simulink model "WindEmulatorDriveSim"  (R2021a)
settings: Solver=FixedStepDiscrete  StartTime=0.0  StopTime=inf  FixedStep=0.002  RelTol=1e-3
values from neighbouring files (symbols this model uses):
  ctrlModeSpeed = logical(false)    [initStep4.m]
  ctrlModeTorque = logical(true)    [initStep4.m]
  StatusWord = bitset(StatusWord,16)    [VFD_StatusWord.m]
undefined symbols (not defined in the file or in its folder): Gen_REF2_Max, Gen_SpeedScaling, Motor_SpeedScaling, Motor_TorqueScaling
libraries: slrealtimeethercatlib x21, simulink x4
settings Model: SimulationMode=external  Creator=SWEPT  LastModifiedBy=Johannes
settings SolverCC: ConcurrentTasks=on  PositivePriorityOrder=on
settings OptimizationCC: BlockReduction=off  OptimizeBlockIOStorage=off
settings DebuggingCC: TasksWithSamePriorityMsg=none
settings HardwareCC: ProdBitPerLong=64  ProdLongLongMode=on  ProdHWDeviceType=Intel->x86-64 (Linux 64)
settings RTWCC: Description=Simulink Real-Time  SystemTargetFile=slrealtime.tlc  TemplateMakefile=slrealtime_default_tmf  RTWVerbose=off  Toolchain=Simulink Real-Time Toolchain  BuildConfiguration=Faster Runs  CodeExecutionProfiling=on  TargetLang=C++

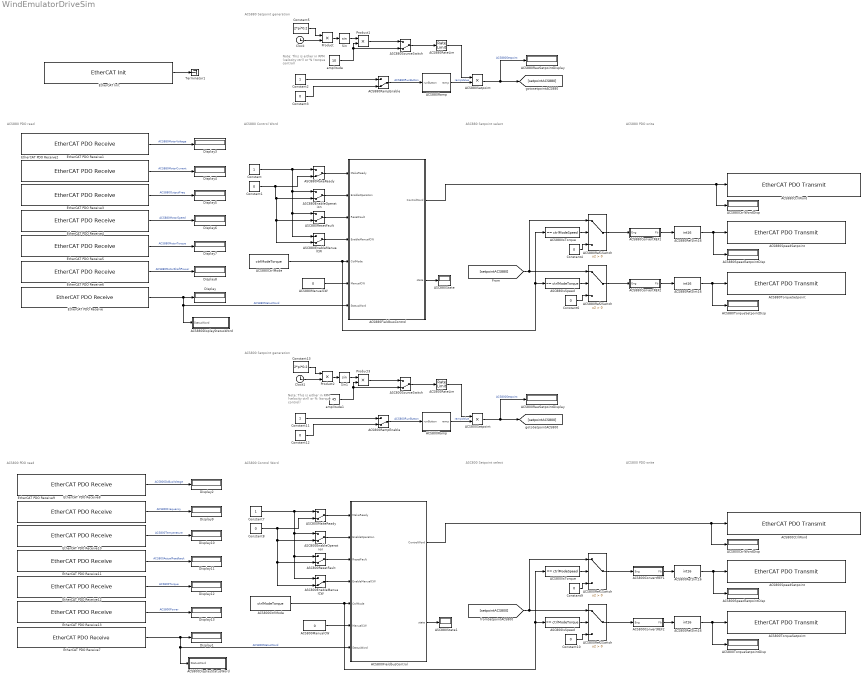
== system WindEmulatorDriveSim ==
  note: ACS880 Setpoint generation
  note: ACS880 PDO write
  note: ASC880 Setpoint select
  note: Note: This is either in RPM (velocity ctrl) or % (torque control)
  note: ACS880 Control Word
  note: ACS880 PDO read
  note: ACS800 PDO read
  note: ACS800 Control Word
  note: ASC800 Setpoint select
  note: ACS800 PDO write
  note: ACS800 Setpoint generation
  note: Note: This is either in RPM (velocity ctrl) or % (torque control)
  ACS800ConvertREF1 : Subsystem  mask{EngineeringValue=Gen_SpeedScaling, FieldbusValue=20000}
      mask prompts: EngineeringValue "Engineering units nominal value:"; FieldbusValue "Fieldbus nominal value:"
  ACS800ConvertREF2 : Subsystem  mask{EngineeringValue=Gen_REF2_Max, FieldbusValue=10000}
      mask prompts: EngineeringValue "Engineering units nominal value:"; FieldbusValue "Fieldbus nominal value:"
  ACS800CtrlMode : Constant  Value=ctrlModeTorque  OutDataTypeStr=boolean
  ACS800CtrlWord : slrealtimeethercatlib/EtherCAT PDO Transmit  Priority=3  sig_name=Drive 2 (RECA-01 r2.07 and ACS800).RxPDO 1.ControlWord (Transparent)  sig_offset=384  sig_type=uint16  type_size=16  sig_dim=1  device_id=0  sample_time=0.002000
      settings: SourceProductBaseCode=XP
  ACS800CtrlWordDisp : Display
  ACS800DisplayStatusWord : Subsystem
  ACS800FieldbusControl : Subsystem
  ACS800IsTorque : simulink/Logic and Bit Operations/Compare To Constant  relop===  const=ctrlModeSpeed  OutDataTypeStr=boolean
  ACS800ManualCW : Constant  Value=0  OutDataTypeStr=uint16
  ACS800Ramp : Stateflow chart  TreatAsAtomicUnit=on
  ACS800RampEnable : ManualSwitch  CurrentSetting=0
  ACS800RateLim : RateLimiter  RisingSlewLimit=10000  FallingSlewLimit=-10000  SampleTimeMode=inherited
  ACS800RawSetpointDisplay : Display
  ACS800Ref1Int16 : DataTypeConversion  OutDataTypeStr=int16
  ACS800Ref1Switch : Switch  Criteria=u2 > Threshold
  ACS800Ref2Int16 : DataTypeConversion  OutDataTypeStr=int16
  ACS800Ref2Switch : Switch  Criteria=u2 > Threshold
  ACS800Setpoint : Product
  ACS800SpeedSetpoint : slrealtimeethercatlib/EtherCAT PDO Transmit  Priority=3  sig_name=Drive 2 (RECA-01 r2.07 and ACS800).RxPDO 1.REF1 (Speed)  sig_offset=400  sig_type=int16  type_size=16  sig_dim=1  device_id=0  sample_time=0.002000
      settings: SourceProductBaseCode=XP
  ACS800SpeedSetpointDisp : Display
  ACS800TorqueSetpoint : slrealtimeethercatlib/EtherCAT PDO Transmit  Priority=3  sig_name=Drive 2 (RECA-01 r2.07 and ACS800).RxPDO 1.REF2 (Torque)  sig_offset=416  sig_type=int16  type_size=16  sig_dim=1  device_id=0  sample_time=0.002000
      settings: SourceProductBaseCode=XP
  ACS800TorqueSetpointDisp : Display
  ACS880ConvertREF1 : Subsystem  mask{EngineeringValue=Motor_SpeedScaling, FieldbusValue=20000}
      mask prompts: EngineeringValue "Engineering units nominal value:"; FieldbusValue "Fieldbus nominal value:"
  ACS880ConvertREF2 : Subsystem  mask{EngineeringValue=Motor_TorqueScaling, FieldbusValue=10000}
      mask prompts: EngineeringValue "Engineering units nominal value:"; FieldbusValue "Fieldbus nominal value:"
  ACS880CtrlMode : Constant  Value=ctrlModeTorque  OutDataTypeStr=boolean
  ACS880CtrlWord : slrealtimeethercatlib/EtherCAT PDO Transmit  Priority=3  sig_name=Drive 1 (FECA-01 r1.31 and ACS880).RxPDO 1.ABB Drives Control Word  sig_offset=208  sig_type=uint16  type_size=16  sig_dim=1  device_id=0  sample_time=0.002000
      settings: SourceProductBaseCode=XP
  ACS880CtrlWordDisp : Display
  ACS880DisplayStatusWord : Subsystem
  ACS880FieldbusControl : Subsystem
  ACS880IsTorque : simulink/Logic and Bit Operations/Compare To Constant  relop===  const=ctrlModeSpeed  OutDataTypeStr=boolean
  ACS880ManualCW : Constant  Value=0  OutDataTypeStr=uint16
  ACS880Ramp : Stateflow chart  TreatAsAtomicUnit=on
  ACS880RampEnable : ManualSwitch  CurrentSetting=0
  ACS880RateLim : RateLimiter  RisingSlewLimit=10000  FallingSlewLimit=-10000  SampleTimeMode=inherited
  ACS880RawSetpointDisplay : Display
  ACS880Ref1Int16 : DataTypeConversion  OutDataTypeStr=int16
  ACS880Ref1Switch : Switch  Criteria=u2 > Threshold
  ACS880Ref2Int16 : DataTypeConversion  OutDataTypeStr=int16
  ACS880Ref2Switch : Switch  Criteria=u2 > Threshold
  ACS880Setpoint : Product
  ACS880SpeedSetpoint : slrealtimeethercatlib/EtherCAT PDO Transmit  Priority=3  sig_name=Drive 1 (FECA-01 r1.31 and ACS880).RxPDO 1.ABB Drives REF1  sig_offset=224  sig_type=int16  type_size=16  sig_dim=1  device_id=0  sample_time=0.002000
      settings: SourceProductBaseCode=XP
  ACS880SpeedSetpointDisp : Display
  ACS880TorqueSetpoint : slrealtimeethercatlib/EtherCAT PDO Transmit  Priority=3  sig_name=Drive 1 (FECA-01 r1.31 and ACS880).RxPDO 1.ABB Drives REF2  sig_offset=240  sig_type=int16  type_size=16  sig_dim=1  device_id=0  sample_time=0.002000
      settings: SourceProductBaseCode=XP
  ACS880TorqueSetpointDisp : Display
  ASC800EnableManualCW : ManualSwitch  CurrentSetting=0
  ASC800EnableOperation : ManualSwitch  CurrentSetting=0
  ASC800IsSpeed : simulink/Logic and Bit Operations/Compare To Constant  relop===  const=ctrlModeTorque  OutDataTypeStr=boolean
  ASC800MakeReady : ManualSwitch  CurrentSetting=0
  ASC800ResetFault : ManualSwitch  CurrentSetting=0
  ASC800SourceSwitch : ManualSwitch  CurrentSetting=0
  ASC880EnableManualCW : ManualSwitch  CurrentSetting=0
  ASC880EnableOperation : ManualSwitch  CurrentSetting=0
  ASC880IsSpeed : simulink/Logic and Bit Operations/Compare To Constant  relop===  const=ctrlModeTorque  OutDataTypeStr=boolean
  ASC880MakeReady : ManualSwitch  CurrentSetting=0
  ASC880ResetFault : ManualSwitch  CurrentSetting=0
  ASC880SourceSwitch : ManualSwitch  CurrentSetting=0
  ASC880State : Display
  ASC880State1 : Display
  Clock : Clock
  Clock1 : Clock
  Constant{,2,7,11} (4 alike) : Constant
  Constant{1,3..4,6,8..10,12} (8 alike) : Constant  Value=0
  Constant13 : Constant  Value=2*pi*0.2
  Constant5 : Constant  Value=2*pi*0.2
  Display{,1..13} (14 alike) : Display
  EtherCAT Init : slrealtimeethercatlib/EtherCAT Init  Priority=0  config_file=D:\src\sandia\ptoTest\WindEmulatorFiles\ethercat\WindTurbineEmulator-03-24-2022.xml  device_id=0  pci_bus=0  pci_slot=0  pci_function=0  portnum=1  initstate=2  dctuning=0  enaDebug=0  enaDC=on  errLink=off  masterDbg=off  stateChgDbg=off  baseClock=off  masterCfg=off  logFile='c:\dbglog.txt'  sample_time=0.002000  DCMode=0
      settings: SourceProductBaseCode=XP
  EtherCAT PDO Receive : slrealtimeethercatlib/EtherCAT PDO Receive  Priority=2  sig_name=Drive 1 (FECA-01 r1.31 and ACS880).TxPDO 1.ABB Drives Status Word  sig_offset=208  sig_type=uint16  type_size=16  sig_dim=1  device_id=0  sample_time=0.002000
      settings: SourceProductBaseCode=XP
  EtherCAT PDO Receive1 : slrealtimeethercatlib/EtherCAT PDO Receive  Priority=2  sig_name=Drive 1 (FECA-01 r1.31 and ACS880).TxPDO 6.Calculated motor voltage  sig_offset=304  sig_type=int16  type_size=16  sig_dim=1  device_id=0  sample_time=0.002000
      settings: SourceProductBaseCode=XP
  EtherCAT PDO Receive10 : slrealtimeethercatlib/EtherCAT PDO Receive  Priority=2  sig_name=Drive 2 (RECA-01 r2.07 and ACS800).TxPDO 1.Converter Temperature  sig_offset=496  sig_type=int16  type_size=16  sig_dim=1  device_id=0  sample_time=0.002000
      settings: SourceProductBaseCode=XP
  EtherCAT PDO Receive11 : slrealtimeethercatlib/EtherCAT PDO Receive  Priority=2  sig_name=Drive 2 (RECA-01 r2.07 and ACS800).TxPDO 1.Actual Feedback (Transparent)  sig_offset=400  sig_type=int16  type_size=16  sig_dim=1  device_id=0  sample_time=0.002000
      settings: SourceProductBaseCode=XP
  EtherCAT PDO Receive12 : slrealtimeethercatlib/EtherCAT PDO Receive  Priority=2  sig_name=Drive 2 (RECA-01 r2.07 and ACS800).TxPDO 1.Torque  sig_offset=432  sig_type=int16  type_size=16  sig_dim=1  device_id=0  sample_time=0.002000
      settings: SourceProductBaseCode=XP
  EtherCAT PDO Receive13 : slrealtimeethercatlib/EtherCAT PDO Receive  Priority=2  sig_name=Drive 2 (RECA-01 r2.07 and ACS800).TxPDO 1.Power  sig_offset=448  sig_type=int16  type_size=16  sig_dim=1  device_id=0  sample_time=0.002000
      settings: SourceProductBaseCode=XP
  EtherCAT PDO Receive2 : slrealtimeethercatlib/EtherCAT PDO Receive  Priority=2  sig_name=Drive 1 (FECA-01 r1.31 and ACS880).TxPDO 6.Measured motor current  sig_offset=288  sig_type=int16  type_size=16  sig_dim=1  device_id=0  sample_time=0.002000
      settings: SourceProductBaseCode=XP
  EtherCAT PDO Receive3 : slrealtimeethercatlib/EtherCAT PDO Receive  Priority=2  sig_name=Drive 1 (FECA-01 r1.31 and ACS880).TxPDO 6.Estimated output frequency  sig_offset=272  sig_type=int16  type_size=16  sig_dim=1  device_id=0  sample_time=0.002000
      settings: SourceProductBaseCode=XP
  EtherCAT PDO Receive4 : slrealtimeethercatlib/EtherCAT PDO Receive  Priority=2  sig_name=Drive 1 (FECA-01 r1.31 and ACS880).TxPDO 6.Motor speed used  sig_offset=256  sig_type=int16  type_size=16  sig_dim=1  device_id=0  sample_time=0.002000
      settings: SourceProductBaseCode=XP
  EtherCAT PDO Receive5 : slrealtimeethercatlib/EtherCAT PDO Receive  Priority=2  sig_name=Drive 1 (FECA-01 r1.31 and ACS880).TxPDO 6.Motor torque  sig_offset=320  sig_type=int16  type_size=16  sig_dim=1  device_id=0  sample_time=0.002000
      settings: SourceProductBaseCode=XP
  EtherCAT PDO Receive6 : slrealtimeethercatlib/EtherCAT PDO Receive  Priority=2  sig_name=Drive 1 (FECA-01 r1.31 and ACS880).TxPDO 6.Estimated motor shaft power  sig_offset=336  sig_type=int16  type_size=16  sig_dim=1  device_id=0  sample_time=0.002000
      settings: SourceProductBaseCode=XP
  EtherCAT PDO Receive7 : slrealtimeethercatlib/EtherCAT PDO Receive  Priority=2  sig_name=Drive 2 (RECA-01 r2.07 and ACS800).TxPDO 1.Main StatusWord (Transparent)  sig_offset=384  sig_type=uint16  type_size=16  sig_dim=1  device_id=0  sample_time=0.002000
      settings: SourceProductBaseCode=XP
  EtherCAT PDO Receive8 : slrealtimeethercatlib/EtherCAT PDO Receive  Priority=2  sig_name=Drive 2 (RECA-01 r2.07 and ACS800).TxPDO 1.DC Bus Voltage  sig_offset=480  sig_type=int16  type_size=16  sig_dim=1  device_id=0  sample_time=0.002000
      settings: SourceProductBaseCode=XP
  EtherCAT PDO Receive9 : slrealtimeethercatlib/EtherCAT PDO Receive  Priority=2  sig_name=Drive 2 (RECA-01 r2.07 and ACS800).TxPDO 1.Frequency  sig_offset=464  sig_type=int16  type_size=16  sig_dim=1  device_id=0  sample_time=0.002000
      settings: SourceProductBaseCode=XP
  Product{,1..3} (4 alike) : Product
  Sin : Trigonometry
  Sin1 : Trigonometry
  Terminator1 : Terminator
  amplitude : Constant  Value=10
  amplitude1 : Constant  Value=45
  wires:
  EtherCAT Init/1 -> Terminator1/1
  ASC880EnableOperation/1 -> ACS880FieldbusControl/2(EnableOperation)
  ACS880ManualCW/1 -> ACS880FieldbusControl/6(ManualCW)
  ASC880ResetFault/1 -> ACS880FieldbusControl/3(ResetFault)
  ASC880MakeReady/1 -> ACS880FieldbusControl/1(MakeReady)
  ASC880EnableManualCW/1 -> ACS880FieldbusControl/4(EnableManualCW)
  Constant1/1 -> ASC880EnableManualCW/2, ASC880ResetFault/2, ASC880EnableOperation/2, ASC880MakeReady/2
  Constant/1 -> ASC880EnableManualCW/1, ASC880ResetFault/1, ASC880EnableOperation/1, ASC880MakeReady/1
  ACS880FieldbusControl/2(state) -> ASC880State/1
  EtherCAT PDO Receive1/1 -> Display3/1  "ACS880MotorVoltage"
  EtherCAT PDO Receive2/1 -> Display4/1  "ACS880MotorCurrent"
  EtherCAT PDO Receive3/1 -> Display5/1  "ACS880OutputFreq"
  EtherCAT PDO Receive4/1 -> Display6/1  "ACS880MotorSpeed"
  EtherCAT PDO Receive5/1 -> Display7/1  "ACS880MotorTorque"
  EtherCAT PDO Receive6/1 -> Display8/1  "ACS880MotorShaftPower"
  ACS880RampEnable/1 -> ACS880Ramp/1(runButton)  "ACS880RunButton"
  Constant3/1 -> ACS880RampEnable/2
  Constant2/1 -> ACS880RampEnable/1
  ACS880Ramp/1(ramp) -> ACS880Setpoint/2  "rampValue"
  Clock/1 -> Product/2
  Product/1 -> Sin/1
  Constant5/1 -> Product/1
  ACS880Setpoint/1 -> [setpointACS880], ACS880RawSetpointDisplay/1  "ACS880Setpoint"
  ACS880RateLim/1 -> ACS880Setpoint/1
  ACS880ConvertREF1/1(Fb) -> ACS880Ref1Int16/1
  ACS880Ref1Int16/1 -> ACS880SpeedSetpointDisp/1, ACS880SpeedSetpoint/1
  ACS880Ref2Int16/1 -> ACS880TorqueSetpoint/1, ACS880TorqueSetpointDisp/1
  ACS880ConvertREF2/1(Fb) -> ACS880Ref2Int16/1
  ACS880CtrlMode/1 -> ACS880FieldbusControl/5(CtrlMode), ACS880IsTorque/1, ASC880IsSpeed/1
  EtherCAT PDO Receive/1 -> ACS880DisplayStatusWord/1(StatusWord), ACS880FieldbusControl/7(StatusWord), Display/1  "ACS880StatusWord"
  ACS880IsTorque/1 -> ACS880Ref1Switch/2
  [setpointACS880] -> ACS880Ref1Switch/1, ACS880Ref2Switch/1
  Constant4/1 -> ACS880Ref1Switch/3
  ASC880IsSpeed/1 -> ACS880Ref2Switch/2
  Constant6/1 -> ACS880Ref2Switch/3
  ACS880FieldbusControl/1(ControlWord) -> ACS880CtrlWordDisp/1, ACS880CtrlWord/1
  ACS880Ref1Switch/1 -> ACS880ConvertREF1/1(Eng)
  ACS880Ref2Switch/1 -> ACS880ConvertREF2/1(Eng)
  Sin/1 -> Product1/1
  amplitude/1 -> Product1/2, ASC880SourceSwitch/2
  Product1/1 -> ASC880SourceSwitch/1
  ASC880SourceSwitch/1 -> ACS880RateLim/1
  EtherCAT PDO Receive13/1 -> Display13/1  "ACS800Power"
  EtherCAT PDO Receive11/1 -> Display11/1  "ACS800ActualFeedback"
  EtherCAT PDO Receive9/1 -> Display9/1  "ACS800Frequency"
  EtherCAT PDO Receive12/1 -> Display12/1  "ACS800Torque"
  EtherCAT PDO Receive10/1 -> Display10/1  "ACS800Temperature"
  EtherCAT PDO Receive8/1 -> Display2/1  "ACS800DcBusVoltage"
  ASC800EnableOperation/1 -> ACS800FieldbusControl/2(EnableOperation)
  ASC800ResetFault/1 -> ACS800FieldbusControl/3(ResetFault)
  ACS800ManualCW/1 -> ACS800FieldbusControl/6(ManualCW)
  EtherCAT PDO Receive7/1 -> ACS800FieldbusControl/7(StatusWord), ACS800DisplayStatusWord/1(StatusWord), Display1/1  "ACS800StatusWord"
  Constant7/1 -> ASC800EnableManualCW/1, ASC800ResetFault/1, ASC800EnableOperation/1, ASC800MakeReady/1
  ACS800FieldbusControl/2(state) -> ASC880State1/1
  Constant8/1 -> ASC800EnableManualCW/2, ASC800ResetFault/2, ASC800EnableOperation/2, ASC800MakeReady/2
  ASC800MakeReady/1 -> ACS800FieldbusControl/1(MakeReady)
  ASC800EnableManualCW/1 -> ACS800FieldbusControl/4(EnableManualCW)
  Constant10/1 -> ACS800Ref2Switch/3
  ASC800IsSpeed/1 -> ACS800Ref2Switch/2
  Constant9/1 -> ACS800Ref1Switch/3
  [setpointACS800] -> ACS800Ref2Switch/1, ACS800Ref1Switch/1
  ACS800IsTorque/1 -> ACS800Ref1Switch/2
  ACS800CtrlMode/1 -> ASC800IsSpeed/1, ACS800IsTorque/1, ACS800FieldbusControl/5(CtrlMode)
  ACS800ConvertREF2/1(Fb) -> ACS800Ref2Int16/1
  ACS800Ref2Int16/1 -> ACS800TorqueSetpointDisp/1, ACS800TorqueSetpoint/1
  ACS800Ref1Int16/1 -> ACS800SpeedSetpoint/1, ACS800SpeedSetpointDisp/1
  ACS800ConvertREF1/1(Fb) -> ACS800Ref1Int16/1
  ACS800FieldbusControl/1(ControlWord) -> ACS800CtrlWordDisp/1, ACS800CtrlWord/1
  ACS800Ref1Switch/1 -> ACS800ConvertREF1/1(Eng)
  ACS800Ref2Switch/1 -> ACS800ConvertREF2/1(Eng)
  ASC800SourceSwitch/1 -> ACS800RateLim/1
  Product3/1 -> ASC800SourceSwitch/1
  amplitude1/1 -> ASC800SourceSwitch/2, Product3/2
  Sin1/1 -> Product3/1
  ACS800RateLim/1 -> ACS800Setpoint/1
  ACS800Setpoint/1 -> ACS800RawSetpointDisplay/1, [setpointACS800]  "ACS800Setpoint"
  Constant13/1 -> Product2/1
  Product2/1 -> Sin1/1
  Clock1/1 -> Product2/2
  ACS800Ramp/1(ramp) -> ACS800Setpoint/2  "rampValue"
  Constant11/1 -> ACS800RampEnable/1
  Constant12/1 -> ACS800RampEnable/2
  ACS800RampEnable/1 -> ACS800Ramp/1(runButton)  "ACS800RunButton"

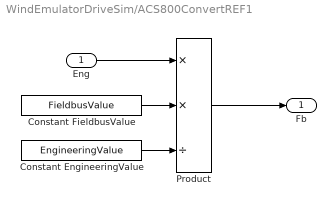
== system WindEmulatorDriveSim/ACS800ConvertREF1 ==
  Eng : Inport
  Constant EngineeringValue : Constant  Value=EngineeringValue
  Constant FieldbusValue : Constant  Value=FieldbusValue
  Product : Product  Inputs=**/
  Fb : Outport
  wires:
  Constant EngineeringValue/1 -> Product/3
  Constant FieldbusValue/1 -> Product/2
  Eng/1 -> Product/1
  Product/1 -> Fb/1

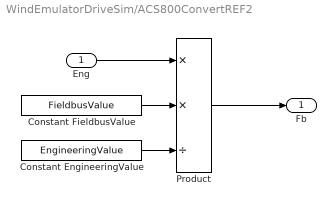
== system WindEmulatorDriveSim/ACS800ConvertREF2 ==
  Eng : Inport
  Constant EngineeringValue : Constant  Value=EngineeringValue
  Constant FieldbusValue : Constant  Value=FieldbusValue
  Product : Product  Inputs=**/
  Fb : Outport
  wires:
  Constant EngineeringValue/1 -> Product/3
  Constant FieldbusValue/1 -> Product/2
  Eng/1 -> Product/1
  Product/1 -> Fb/1

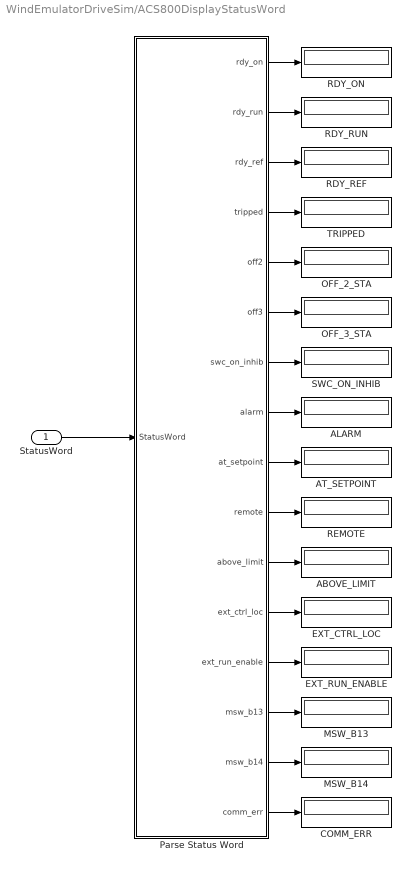
== system WindEmulatorDriveSim/ACS800DisplayStatusWord ==
  StatusWord : Inport
  ABOVE_LIMIT : Display
  ALARM : Display
  AT_SETPOINT : Display
  COMM_ERR : Display
  EXT_CTRL_LOC : Display
  EXT_RUN_ENABLE : Display
  MSW_B13 : Display
  MSW_B14 : Display
  OFF_2_STA : Display
  OFF_3_STA : Display
  Parse Status Word : MATLAB Function  TreatAsAtomicUnit=on
  RDY_ON : Display
  RDY_REF : Display
  RDY_RUN : Display
  REMOTE : Display
  SWC_ON_INHIB : Display
  TRIPPED : Display
  wires:
  Parse Status Word/11(above_limit) -> ABOVE_LIMIT/1
  Parse Status Word/3(rdy_ref) -> RDY_REF/1
  Parse Status Word/16(comm_err) -> COMM_ERR/1
  Parse Status Word/15(msw_b14) -> MSW_B14/1
  Parse Status Word/14(msw_b13) -> MSW_B13/1
  Parse Status Word/8(alarm) -> ALARM/1
  Parse Status Word/2(rdy_run) -> RDY_RUN/1
  Parse Status Word/5(off2) -> OFF_2_STA/1
  Parse Status Word/12(ext_ctrl_loc) -> EXT_CTRL_LOC/1
  Parse Status Word/4(tripped) -> TRIPPED/1
  Parse Status Word/6(off3) -> OFF_3_STA/1
  Parse Status Word/1(rdy_on) -> RDY_ON/1
  Parse Status Word/9(at_setpoint) -> AT_SETPOINT/1
  Parse Status Word/7(swc_on_inhib) -> SWC_ON_INHIB/1
  Parse Status Word/13(ext_run_enable) -> EXT_RUN_ENABLE/1
  Parse Status Word/10(remote) -> REMOTE/1
  StatusWord/1 -> Parse Status Word/1(StatusWord)

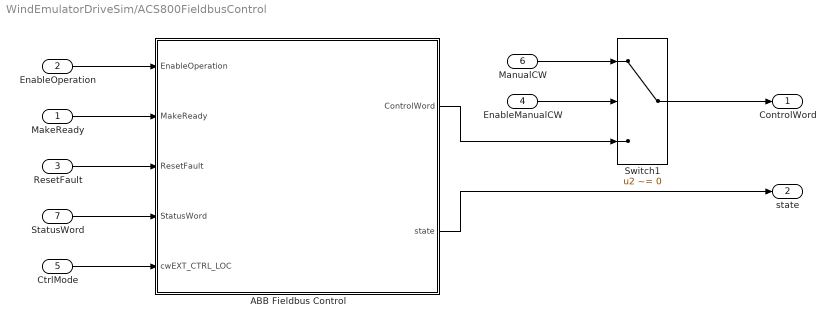
== system WindEmulatorDriveSim/ACS800FieldbusControl ==
  MakeReady : Inport
  EnableOperation : Inport  Port=2
  ResetFault : Inport  Port=3
  EnableManualCW : Inport  Port=4
  CtrlMode : Inport  Port=5
  ManualCW : Inport  Port=6  OutDataTypeStr=uint16
  StatusWord : Inport  Port=7
  ABB Fieldbus Control : Stateflow chart  TreatAsAtomicUnit=on
  Switch1 : Switch  Criteria=u2 ~= 0
  ControlWord : Outport
  state : Outport  Port=2
  wires:
  EnableOperation/1 -> ABB Fieldbus Control/1(EnableOperation)
  ManualCW/1 -> Switch1/1
  MakeReady/1 -> ABB Fieldbus Control/2(MakeReady)
  ABB Fieldbus Control/1(ControlWord) -> Switch1/3
  ResetFault/1 -> ABB Fieldbus Control/3(ResetFault)
  Switch1/1 -> ControlWord/1
  EnableManualCW/1 -> Switch1/2
  StatusWord/1 -> ABB Fieldbus Control/4(StatusWord)
  ABB Fieldbus Control/2(state) -> state/1
  CtrlMode/1 -> ABB Fieldbus Control/5(cwEXT_CTRL_LOC)

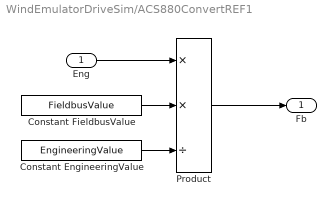
== system WindEmulatorDriveSim/ACS880ConvertREF1 ==
  Eng : Inport
  Constant EngineeringValue : Constant  Value=EngineeringValue
  Constant FieldbusValue : Constant  Value=FieldbusValue
  Product : Product  Inputs=**/
  Fb : Outport
  wires:
  Product/1 -> Fb/1
  Eng/1 -> Product/1
  Constant FieldbusValue/1 -> Product/2
  Constant EngineeringValue/1 -> Product/3

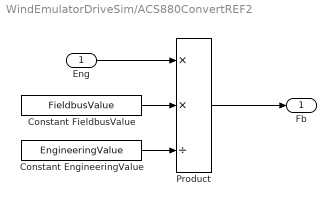
== system WindEmulatorDriveSim/ACS880ConvertREF2 ==
  Eng : Inport
  Constant EngineeringValue : Constant  Value=EngineeringValue
  Constant FieldbusValue : Constant  Value=FieldbusValue
  Product : Product  Inputs=**/
  Fb : Outport
  wires:
  Product/1 -> Fb/1
  Eng/1 -> Product/1
  Constant FieldbusValue/1 -> Product/2
  Constant EngineeringValue/1 -> Product/3

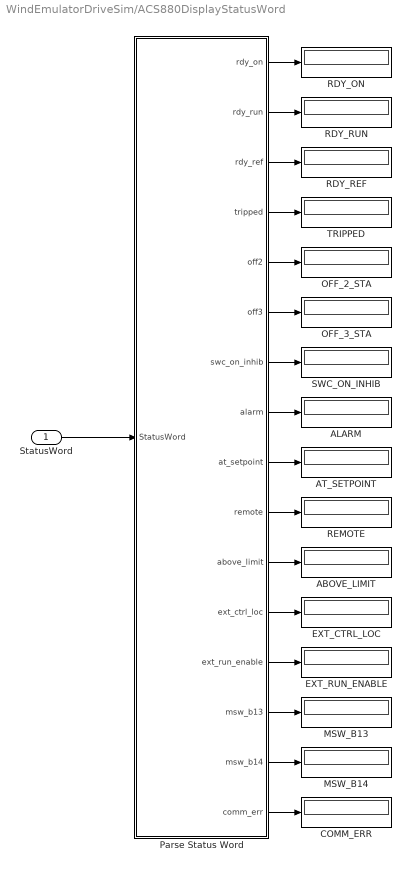
== system WindEmulatorDriveSim/ACS880DisplayStatusWord ==
  StatusWord : Inport
  ABOVE_LIMIT : Display
  ALARM : Display
  AT_SETPOINT : Display
  COMM_ERR : Display
  EXT_CTRL_LOC : Display
  EXT_RUN_ENABLE : Display
  MSW_B13 : Display
  MSW_B14 : Display
  OFF_2_STA : Display
  OFF_3_STA : Display
  Parse Status Word : MATLAB Function  TreatAsAtomicUnit=on
  RDY_ON : Display
  RDY_REF : Display
  RDY_RUN : Display
  REMOTE : Display
  SWC_ON_INHIB : Display
  TRIPPED : Display
  wires:
  Parse Status Word/11(above_limit) -> ABOVE_LIMIT/1
  Parse Status Word/3(rdy_ref) -> RDY_REF/1
  Parse Status Word/16(comm_err) -> COMM_ERR/1
  Parse Status Word/15(msw_b14) -> MSW_B14/1
  Parse Status Word/14(msw_b13) -> MSW_B13/1
  Parse Status Word/8(alarm) -> ALARM/1
  Parse Status Word/2(rdy_run) -> RDY_RUN/1
  Parse Status Word/5(off2) -> OFF_2_STA/1
  Parse Status Word/12(ext_ctrl_loc) -> EXT_CTRL_LOC/1
  Parse Status Word/4(tripped) -> TRIPPED/1
  Parse Status Word/6(off3) -> OFF_3_STA/1
  Parse Status Word/1(rdy_on) -> RDY_ON/1
  Parse Status Word/9(at_setpoint) -> AT_SETPOINT/1
  Parse Status Word/7(swc_on_inhib) -> SWC_ON_INHIB/1
  Parse Status Word/13(ext_run_enable) -> EXT_RUN_ENABLE/1
  Parse Status Word/10(remote) -> REMOTE/1
  StatusWord/1 -> Parse Status Word/1(StatusWord)

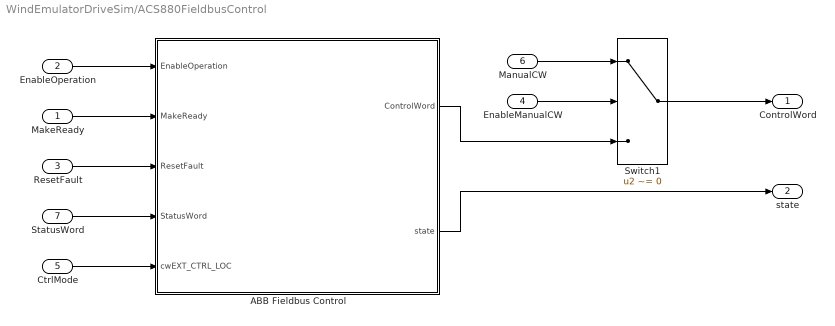
== system WindEmulatorDriveSim/ACS880FieldbusControl ==
  MakeReady : Inport
  EnableOperation : Inport  Port=2
  ResetFault : Inport  Port=3
  EnableManualCW : Inport  Port=4
  CtrlMode : Inport  Port=5
  ManualCW : Inport  Port=6  OutDataTypeStr=uint16
  StatusWord : Inport  Port=7
  ABB Fieldbus Control : Stateflow chart  TreatAsAtomicUnit=on
  Switch1 : Switch  Criteria=u2 ~= 0
  ControlWord : Outport
  state : Outport  Port=2
  wires:
  EnableOperation/1 -> ABB Fieldbus Control/1(EnableOperation)
  ManualCW/1 -> Switch1/1
  MakeReady/1 -> ABB Fieldbus Control/2(MakeReady)
  ABB Fieldbus Control/1(ControlWord) -> Switch1/3
  ResetFault/1 -> ABB Fieldbus Control/3(ResetFault)
  Switch1/1 -> ControlWord/1
  EnableManualCW/1 -> Switch1/2
  StatusWord/1 -> ABB Fieldbus Control/4(StatusWord)
  ABB Fieldbus Control/2(state) -> state/1
  CtrlMode/1 -> ABB Fieldbus Control/5(cwEXT_CTRL_LOC)

== matlab function WindEmulatorDriveSim/ACS880DisplayStatusWord/Parse Status Word ==
  data: StatusWord input; rdy_on output; rdy_run output; rdy_ref output; tripped output; off2 output; off3 output; swc_on_inhib output; alarm output; at_setpoint output; remote output; above_limit output; ext_ctrl_loc output; ext_run_enable output; msw_b13 output; msw_b14 output; comm_err output
function [rdy_on,rdy_run,rdy_ref,tripped,off2,off3,swc_on_inhib,alarm,...
    at_setpoint,remote,above_limit,ext_ctrl_loc,ext_run_enable,...
    msw_b13,msw_b14,comm_err]  = fcn(StatusWord)

SW = VFD_StatusWord(StatusWord);
rdy_on = SW.RDY_ON;
rdy_run = SW.RDY_RUN;
rdy_ref = SW.RDY_REF;
tripped = SW.TRIPPED;
off2 = SW.OFF_2_STA;
off3 = SW.OFF_3_STA;
swc_on_inhib = SW.SWC_ON_INHIB;
alarm = SW.ALARM;
at_setpoint = SW.AT_SETPOINT;
remote = SW.REMOTE;
above_limit = SW.ABOVE_LIMIT;
ext_ctrl_loc = SW.EXT_CTRL_LOC;
ext_run_enable = SW.EXT_RUN_ENABLE;
msw_b13 = SW.MSW_B13;
msw_b14 = SW.MSW_B14;
comm_err = SW.COMM_ERR;

== matlab function WindEmulatorDriveSim/ACS800DisplayStatusWord/Parse Status Word ==
  data: StatusWord input; rdy_on output; rdy_run output; rdy_ref output; tripped output; off2 output; off3 output; swc_on_inhib output; alarm output; at_setpoint output; remote output; above_limit output; ext_ctrl_loc output; ext_run_enable output; msw_b13 output; msw_b14 output; comm_err output
function [rdy_on,rdy_run,rdy_ref,tripped,off2,off3,swc_on_inhib,alarm,...
    at_setpoint,remote,above_limit,ext_ctrl_loc,ext_run_enable,...
    msw_b13,msw_b14,comm_err]  = fcn(StatusWord)

SW = VFD_StatusWord(StatusWord);
rdy_on = SW.RDY_ON;
rdy_run = SW.RDY_RUN;
rdy_ref = SW.RDY_REF;
tripped = SW.TRIPPED;
off2 = SW.OFF_2_STA;
off3 = SW.OFF_3_STA;
swc_on_inhib = SW.SWC_ON_INHIB;
alarm = SW.ALARM;
at_setpoint = SW.AT_SETPOINT;
remote = SW.REMOTE;
above_limit = SW.ABOVE_LIMIT;
ext_ctrl_loc = SW.EXT_CTRL_LOC;
ext_run_enable = SW.EXT_RUN_ENABLE;
msw_b13 = SW.MSW_B13;
msw_b14 = SW.MSW_B14;
comm_err = SW.COMM_ERR;

== stateflow chart WindEmulatorDriveSim/ACS800FieldbusControl/ABB Fieldbus Control ==
  state UpdateStateMachine [parallel]
    during:
    swParseStatusWord();
    cwRESET = ResetFault;
    settings: executionOrder=1
    state NotReadyToOperate
      entry:
      cwOFF1_CONTROL=0;
      state ReadyToSwitchOn
        during:
        state=2
      state NotReadyToSwitchOn
        during:
        state=1
      (default) -> NotReadyToSwitchOn
      NotReadyToSwitchOn -> ReadyToSwitchOn : [swRDY_ON==1 && ...
          |  swWARNING==0 && ...
          |  EnableOperation==0]
    state initialize
      entry:
      cwInitialize();
      state=0
    state DelayOFF1
      during:
      state=5
    state ReadyToOperate
      entry:
      cwOFF1_CONTROL=1;
      state OperationDisabled
        during:
        state=3
      state OperationEnabled
        entry:
        cwENABLE_OPERATION=1;
        during:
        state=4
        exit:
        cwENABLE_OPERATION=0;
      OperationDisabled -> OperationEnabled : [swRDY_RUN==1 && ...
          |  EnableOperation==1]
      (default) -> OperationDisabled
      OperationEnabled -> OperationDisabled : [EnableOperation==0]
    initialize -> NotReadyToOperate
    (default) -> initialize
    DelayOFF1 -> NotReadyToSwitchOn : after(100,msec)
    ReadyToSwitchOn -> ReadyToOperate : [MakeReady==1 && ...
        |  swREMOTE==1]
    ReadyToOperate -> DelayOFF1 : [MakeReady==0 || ...
        |  swTRIPPED==1 || ...
        |  swSWC_ON_INHIB==1 || ...
        |  swWARNING==1]
  state UpdateControlWord [parallel]
    during:
    cwBuildControlWord();
    settings: executionOrder=2
  data: EnableOperation input; MakeReady input; swRDY_ON local; swRDY_RUN local; ResetFault input; StatusWord input; swRDY_REF local; swTRIPPED local; swOFF_2_STA local; swOFF_3_STA local; swSWC_ON_INHIB local; swAT_SETPOINT local; swEXT_RUN_ENABLE local; cwOFF2_CONTROL local; cwOFF3_CONTROL local; cwENABLE_OPERATION local; cwRAMP_OUT_ZERO local; cwRAMP_HOLD local; cwRAMP_IN_ZERO local; cwRESET local; cwREMOTE_CMD local; cwOFF1_CONTROL local; swEXT_CTRL_LOC local; swREMOTE local; ControlWord output uint16; swWARNING local; swABOVE_LIMIT local; swMSW_B13 local; swMSW_B14 local; swCOMM_ERR local; state output; cwEXT_CTRL_LOC input
  function cwInitialize:
    | function cwInitialize
    | cwOFF1_CONTROL = 0;
    | cwOFF2_CONTROL = 1;
    | cwOFF3_CONTROL = 1;
    | cwENABLE_OPERATION = 0;
    | cwRAMP_OUT_ZERO = 1;
    | cwRAMP_HOLD = 1;
    | cwRAMP_IN_ZERO = 1;
    | cwRESET = 0;
    | % cwINCHING_1 = 0;
    | % cwINCHING_2 = 0;
    | cwREMOTE_CMD = 1;
    | %cwEXT_CTRL_LOC = 0;
  function cwBuildControlWord:
    | function cwBuildControlWord
    | ControlWord = uint16(0);
    | if cwOFF1_CONTROL
    |     ControlWord = bitset(ControlWord,1);
    | end
    | if cwOFF2_CONTROL
    |     ControlWord = bitset(ControlWord,2);
    | end
    | if cwOFF3_CONTROL
    |     ControlWord = bitset(ControlWord,3);
    | end
    | if cwENABLE_OPERATION
    |     ControlWord = bitset(ControlWord,4);
    | end
    | if cwRAMP_OUT_ZERO
    |     ControlWord = bitset(ControlWord,5);
    | end
    | if cwRAMP_HOLD
    |     ControlWord = bitset(ControlWord,6);
    | end
    | if cwRAMP_IN_ZERO
    |     ControlWord = bitset(ControlWord,7);
    | end
    | if cwRESET
    |     ControlWord = bitset(ControlWord,8);
    | end
    | % if cwINCHING_1
    | %     ControlWord = bitset(ControlWord,9);
    | % end
    | % if cwINCHING_2
    | %     ControlWord = bitset(ControlWord,10);
    | % end
    | if cwREMOTE_CMD
    |     ControlWord = bitset(ControlWord,11);
    | end
    | if cwEXT_CTRL_LOC
    |     ControlWord = bitset(ControlWord,12);
    | end
  function swParseStatusWord:
    | function swParseStatusWord
    | sw = uint16(StatusWord);
    | swRDY_ON = 0;
    | swRDY_RUN = 0;
    | swRDY_REF = 0;
    | swTRIPPED = 0;
    | swOFF_2_STA = 0;
    | swOFF_3_STA = 0;
    | swSWC_ON_INHIB = 0;
    | swWARNING = 0;
    | swAT_SETPOINT = 0;
    | swREMOTE = 0;
    | swABOVE_LIMIT = 0;
    | swEXT_CTRL_LOC = 0;
    | swEXT_RUN_ENABLE = 0;
    | swMSW_B13 = 0;
    | swMSW_B14 = 0;
    | swCOMM_ERR = 0;
    | 
    | if (sw >= 2^15)
    |     swCOMM_ERR = 1;
    |     sw = sw - 2^15;
    | end
    | if (sw >= 2^14)
    |     swMSW_B14 = 1;
    |     sw = sw - 2^14;
    | end
    | if (sw >= 2^13)
    |     swMSW_B13 = 1;
    |     sw = sw - 2^13;
    | end
    | if (sw >= 2^12)
    |     swEXT_RUN_ENABLE = 1;
    |     sw = sw - 2^12;
    | end
    | if (sw >= 2^11)
    |     swEXT_CTRL_LOC = 1;
    |     sw = sw - 2^11;
    | end
    | if (sw >= 2^10)
    |     swABOVE_LIMIT = 1;
    |     sw = sw - 2^10;
    | end
    | if (sw >= 2^9)
    |     swREMOTE = 1;
    |     sw = sw - 2^9;
    | end
    | if (sw >= 2^8)
    |     swAT_SETPOINT = 1;
    |     sw = sw - 2^8;
    | end
    | if (sw >= 2^7)
    |     swWARNING = 1;
    |     sw = sw - 2^7;
    | end
    | if (sw >= 2^6)
    |     swSWC_ON_INHIB = 1;
    |     sw = sw - 2^6;
    | end
    | if (sw >= 2^5)
    |     swOFF_3_STA = 1;
    |     sw = sw - 2^5;
    | end
    | if (sw >= 2^4)
    |     swOFF_2_STA = 1;
    |     sw = sw - 2^4;
    | end
    | if (sw >= 2^3)
    |     swTRIPPED = 1;
    |     sw = sw - 2^3;
    | end
    | if (sw >= 2^2)
    |     swRDY_REF = 1;
    |     sw = sw - 2^2;
    | end
    | if (sw >= 2^1)
    |     swRDY_RUN = 1;
    |     sw = sw - 2^1;
    | end
    | if (sw >= 2^0)
    |     swRDY_ON = 1;
    |     sw = sw - 2^0;
    | end

== stateflow chart WindEmulatorDriveSim/ACS800Ramp ==
  state idle
    during:
    ramp=0
    rampLast=0
  state rampup
    during:
    ramp=min(1,elapsed('sec')/rampTime)
    rampLast = ramp
  state runing
    during:
    ramp=1
    rampLast = ramp
  state rampdown
    during:
    ramp=rampLast-max(0,elapsed('sec')/rampTime)
  (default) -> idle
  rampdown -> idle : [ramp<=0]
  idle -> rampup : [runButton]
  rampup -> rampdown [order 2] : [~runButton]
  rampup -> runing [order 1] : [ramp>=1]
  runing -> rampdown : [~runButton]
  data: ramp output; runButton input; rampLast local; rampTime parameter

== stateflow chart WindEmulatorDriveSim/ACS880Ramp ==
  state idle
    during:
    ramp=0
    rampLast=0
  state rampup
    during:
    ramp=min(1,elapsed('sec')/rampTime)
    rampLast = ramp
  state runing
    during:
    ramp=1
    rampLast = ramp
  state rampdown
    during:
    ramp=rampLast-max(0,elapsed('sec')/rampTime)
  (default) -> idle
  rampdown -> idle : [ramp<=0]
  idle -> rampup : [runButton]
  rampup -> rampdown [order 2] : [~runButton]
  rampup -> runing [order 1] : [ramp>=1]
  runing -> rampdown : [~runButton]
  data: ramp output; runButton input; rampLast local; rampTime parameter

== stateflow chart WindEmulatorDriveSim/ACS880FieldbusControl/ABB Fieldbus Control ==
  state UpdateStateMachine [parallel]
    during:
    swParseStatusWord();
    cwRESET = ResetFault;
    settings: executionOrder=1
    state NotReadyToOperate
      entry:
      cwOFF1_CONTROL=0;
      state ReadyToSwitchOn
        during:
        state=2
      state NotReadyToSwitchOn
        during:
        state=1
      (default) -> NotReadyToSwitchOn
      NotReadyToSwitchOn -> ReadyToSwitchOn : [swRDY_ON==1 && ...
          |  swWARNING==0 && ...
          |  EnableOperation==0]
    state initialize
      entry:
      cwInitialize();
      state=0
    state DelayOFF1
      during:
      state=5
    state ReadyToOperate
      entry:
      cwOFF1_CONTROL=1;
      state OperationDisabled
        during:
        state=3
      state OperationEnabled
        entry:
        cwENABLE_OPERATION=1;
        during:
        state=4
        exit:
        cwENABLE_OPERATION=0;
      OperationDisabled -> OperationEnabled : [swRDY_RUN==1 && ...
          |  EnableOperation==1]
      (default) -> OperationDisabled
      OperationEnabled -> OperationDisabled : [EnableOperation==0]
    initialize -> NotReadyToOperate
    (default) -> initialize
    DelayOFF1 -> NotReadyToSwitchOn : after(100,msec)
    ReadyToSwitchOn -> ReadyToOperate : [MakeReady==1 && ...
        |  swREMOTE==1]
    ReadyToOperate -> DelayOFF1 : [MakeReady==0 || ...
        |  swTRIPPED==1 || ...
        |  swSWC_ON_INHIB==1 || ...
        |  swWARNING==1]
  state UpdateControlWord [parallel]
    during:
    cwBuildControlWord();
    settings: executionOrder=2
  data: EnableOperation input; MakeReady input; swRDY_ON local; swRDY_RUN local; ResetFault input; StatusWord input; swRDY_REF local; swTRIPPED local; swOFF_2_STA local; swOFF_3_STA local; swSWC_ON_INHIB local; swAT_SETPOINT local; swEXT_RUN_ENABLE local; cwOFF2_CONTROL local; cwOFF3_CONTROL local; cwENABLE_OPERATION local; cwRAMP_OUT_ZERO local; cwRAMP_HOLD local; cwRAMP_IN_ZERO local; cwRESET local; cwREMOTE_CMD local; cwOFF1_CONTROL local; swEXT_CTRL_LOC local; swREMOTE local; ControlWord output uint16; swWARNING local; swABOVE_LIMIT local; swMSW_B13 local; swMSW_B14 local; swCOMM_ERR local; state output; cwEXT_CTRL_LOC input
  function cwInitialize:
    | function cwInitialize
    | cwOFF1_CONTROL = 0;
    | cwOFF2_CONTROL = 1;
    | cwOFF3_CONTROL = 1;
    | cwENABLE_OPERATION = 0;
    | cwRAMP_OUT_ZERO = 1;
    | cwRAMP_HOLD = 1;
    | cwRAMP_IN_ZERO = 1;
    | cwRESET = 0;
    | % cwINCHING_1 = 0;
    | % cwINCHING_2 = 0;
    | cwREMOTE_CMD = 1;
    | %cwEXT_CTRL_LOC = 0;
  function cwBuildControlWord:
    | function cwBuildControlWord
    | ControlWord = uint16(0);
    | if cwOFF1_CONTROL
    |     ControlWord = bitset(ControlWord,1);
    | end
    | if cwOFF2_CONTROL
    |     ControlWord = bitset(ControlWord,2);
    | end
    | if cwOFF3_CONTROL
    |     ControlWord = bitset(ControlWord,3);
    | end
    | if cwENABLE_OPERATION
    |     ControlWord = bitset(ControlWord,4);
    | end
    | if cwRAMP_OUT_ZERO
    |     ControlWord = bitset(ControlWord,5);
    | end
    | if cwRAMP_HOLD
    |     ControlWord = bitset(ControlWord,6);
    | end
    | if cwRAMP_IN_ZERO
    |     ControlWord = bitset(ControlWord,7);
    | end
    | if cwRESET
    |     ControlWord = bitset(ControlWord,8);
    | end
    | % if cwINCHING_1
    | %     ControlWord = bitset(ControlWord,9);
    | % end
    | % if cwINCHING_2
    | %     ControlWord = bitset(ControlWord,10);
    | % end
    | if cwREMOTE_CMD
    |     ControlWord = bitset(ControlWord,11);
    | end
    | if cwEXT_CTRL_LOC
    |     ControlWord = bitset(ControlWord,12);
    | end
  function swParseStatusWord:
    | function swParseStatusWord
    | sw = uint16(StatusWord);
    | swRDY_ON = 0;
    | swRDY_RUN = 0;
    | swRDY_REF = 0;
    | swTRIPPED = 0;
    | swOFF_2_STA = 0;
    | swOFF_3_STA = 0;
    | swSWC_ON_INHIB = 0;
    | swWARNING = 0;
    | swAT_SETPOINT = 0;
    | swREMOTE = 0;
    | swABOVE_LIMIT = 0;
    | swEXT_CTRL_LOC = 0;
    | swEXT_RUN_ENABLE = 0;
    | swMSW_B13 = 0;
    | swMSW_B14 = 0;
    | swCOMM_ERR = 0;
    | 
    | if (sw >= 2^15)
    |     swCOMM_ERR = 1;
    |     sw = sw - 2^15;
    | end
    | if (sw >= 2^14)
    |     swMSW_B14 = 1;
    |     sw = sw - 2^14;
    | end
    | if (sw >= 2^13)
    |     swMSW_B13 = 1;
    |     sw = sw - 2^13;
    | end
    | if (sw >= 2^12)
    |     swEXT_RUN_ENABLE = 1;
    |     sw = sw - 2^12;
    | end
    | if (sw >= 2^11)
    |     swEXT_CTRL_LOC = 1;
    |     sw = sw - 2^11;
    | end
    | if (sw >= 2^10)
    |     swABOVE_LIMIT = 1;
    |     sw = sw - 2^10;
    | end
    | if (sw >= 2^9)
    |     swREMOTE = 1;
    |     sw = sw - 2^9;
    | end
    | if (sw >= 2^8)
    |     swAT_SETPOINT = 1;
    |     sw = sw - 2^8;
    | end
    | if (sw >= 2^7)
    |     swWARNING = 1;
    |     sw = sw - 2^7;
    | end
    | if (sw >= 2^6)
    |     swSWC_ON_INHIB = 1;
    |     sw = sw - 2^6;
    | end
    | if (sw >= 2^5)
    |     swOFF_3_STA = 1;
    |     sw = sw - 2^5;
    | end
    | if (sw >= 2^4)
    |     swOFF_2_STA = 1;
    |     sw = sw - 2^4;
    | end
    | if (sw >= 2^3)
    |     swTRIPPED = 1;
    |     sw = sw - 2^3;
    | end
    | if (sw >= 2^2)
    |     swRDY_REF = 1;
    |     sw = sw - 2^2;
    | end
    | if (sw >= 2^1)
    |     swRDY_RUN = 1;
    |     sw = sw - 2^1;
    | end
    | if (sw >= 2^0)
    |     swRDY_ON = 1;
    |     sw = sw - 2^0;
    | end
